simulink model "DynamicTemplate"  (R2018b)
settings: Solver=FixedStepDiscrete  StartTime=0.0  StopTime=Inf  FixedStep=0.001  RelTol=1e-3  EnableMultiTasking=on
undefined symbols (not defined in the file): J1, J2, J3, J4, J5, J6, J7, Motor_Current, Motor_Position, Motor_Velocity, Send_GUIdata
libraries: c280xlib x50, simulink x5, idelinklib_common x1
(part 1 of 5)
settings Model: ExtModeTrigDuration=8  Creator=Administrator  LastModifiedBy=Jeason
settings SolverCC: AutoInsertRateTranBlk=on
settings OptimizationCC: DefaultUnderspecifiedDataType=single  EnhancedBackFolding=on  PassReuseOutputArgsAs=Individual arguments  MaxStackSize=512  OptimizeBlockOrder=speed  DifferentSizesBufferReuse=on  OptimizationCustomize=off
settings DebuggingCC: InheritedTsInSrcMsg=none  MultiTaskDSMMsg=none  ParameterTunabilityLossMsg=error
settings HardwareCC: ProdBitPerChar=16  ProdBitPerInt=16  ProdBitPerPointer=32  ProdBitPerSizeT=32  ProdBitPerPtrDiffT=32  ProdLargestAtomicInteger=Integer  ProdLargestAtomicFloat=None  ProdWordSize=16  ProdLongLongMode=on  ProdHWDeviceType=Texas Instruments->C2000
settings SFSimCC: MATLABDynamicMemAlloc=off
settings RTWCC: SystemTargetFile=ert.tlc  HardwareBoard=TI Delfino F2833x  TemplateMakefile=ert_default_tmf  GenerateReport=on  Toolchain=Texas Instruments Code Composer Studio (C2000)  IncludeHyperlinkInReport=on  LaunchReport=on  GenerateTraceInfo=on  GenerateTraceReport=on  GenerateTraceReportSl=on  GenerateTraceReportSf=on  GenerateTraceReportEml=on
settings CodeAppCC: ForceParamTrailComments=on  IgnoreCustomStorageClasses=off  OperatorAnnotations=on  SimulinkDataObjDesc=on  SFDataObjDesc=on  InsertBlockDesc=on
settings ERTTargetCC: CodeReplacementLibrary=TI C28x

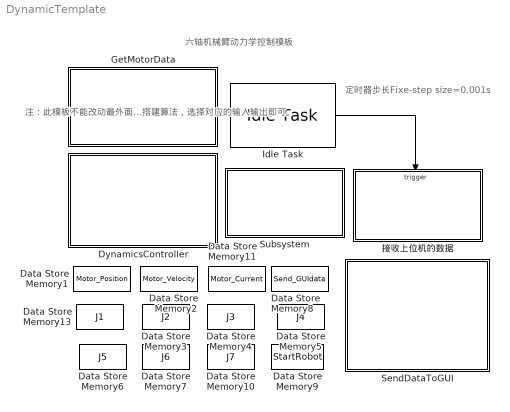
== system DynamicTemplate ==
  note: 六轴机械臂动力学控制模板
  note: 注：此模板不能改动最外面的结构，要做动力学算法只能在动力学计算子系统内部搭建算法，选择对应的输入输出即可。
  note: 定时器步长Fixe-step size=0.001s
  Data Store Memory1 : DataStoreMemory  DataStoreName=Motor_Position  ReadBeforeWriteMsg=warning  WriteAfterWriteMsg=warning  WriteAfterReadMsg=warning  InitialValue=[0 0 0 0 0 0]  ShowAdditionalParam=off  OutDataTypeStr=int32
      settings: RTWStateStorageClass=ExportedGlobal
  Data Store Memory10 : DataStoreMemory  DataStoreName=J7  ReadBeforeWriteMsg=warning  WriteAfterWriteMsg=warning  WriteAfterReadMsg=warning  InitialValue=[0 0 0 0 0 0]  ShowAdditionalParam=off  OutDataTypeStr=double
      settings: RTWStateStorageClass=ExportedGlobal
  Data Store Memory11 : DataStoreMemory  DataStoreName=Motor_Current  ReadBeforeWriteMsg=warning  WriteAfterWriteMsg=warning  WriteAfterReadMsg=warning  InitialValue=[0 0 0 0 0 0]  ShowAdditionalParam=off  OutDataTypeStr=int32
      settings: RTWStateStorageClass=ExportedGlobal
  Data Store Memory13 : DataStoreMemory  DataStoreName=J1  ReadBeforeWriteMsg=warning  WriteAfterWriteMsg=warning  WriteAfterReadMsg=warning  InitialValue=[0 0 0 0 0 0]  ShowAdditionalParam=off  OutDataTypeStr=double
      settings: RTWStateStorageClass=ExportedGlobal
  Data Store Memory2 : DataStoreMemory  DataStoreName=Motor_Velocity  ReadBeforeWriteMsg=warning  WriteAfterWriteMsg=warning  WriteAfterReadMsg=warning  InitialValue=[0 0 0 0 0 0]  ShowAdditionalParam=off  OutDataTypeStr=int32
      settings: RTWStateStorageClass=ExportedGlobal
  Data Store Memory3 : DataStoreMemory  DataStoreName=J2  ReadBeforeWriteMsg=warning  WriteAfterWriteMsg=warning  WriteAfterReadMsg=warning  InitialValue=[0 0 0 0 0 0]  ShowAdditionalParam=off  OutDataTypeStr=double
      settings: RTWStateStorageClass=ExportedGlobal
  Data Store Memory4 : DataStoreMemory  DataStoreName=J3  ReadBeforeWriteMsg=warning  WriteAfterWriteMsg=warning  WriteAfterReadMsg=warning  InitialValue=[0 0 0 0 0 0]  ShowAdditionalParam=off  OutDataTypeStr=double
      settings: RTWStateStorageClass=ExportedGlobal
  Data Store Memory5 : DataStoreMemory  DataStoreName=J4  ReadBeforeWriteMsg=warning  WriteAfterWriteMsg=warning  WriteAfterReadMsg=warning  InitialValue=[0 0 0 0 0 0]  ShowAdditionalParam=off  OutDataTypeStr=double
      settings: RTWStateStorageClass=ExportedGlobal
  Data Store Memory6 : DataStoreMemory  DataStoreName=J5  ReadBeforeWriteMsg=warning  WriteAfterWriteMsg=warning  WriteAfterReadMsg=warning  InitialValue=[0 0 0 0 0 0]  ShowAdditionalParam=off  OutDataTypeStr=double
      settings: RTWStateStorageClass=ExportedGlobal
  Data Store Memory7 : DataStoreMemory  DataStoreName=J6  ReadBeforeWriteMsg=warning  WriteAfterWriteMsg=warning  WriteAfterReadMsg=warning  InitialValue=[0 0 0 0 0 0]  ShowAdditionalParam=off  OutDataTypeStr=double
      settings: RTWStateStorageClass=ExportedGlobal
  Data Store Memory8 : DataStoreMemory  DataStoreName=Send_GUIdata  ReadBeforeWriteMsg=warning  WriteAfterWriteMsg=warning  WriteAfterReadMsg=warning  InitialValue=zeros(1,18)  ShowAdditionalParam=off  OutDataTypeStr=double
      settings: RTWStateStorageClass=ExportedGlobal
  Data Store Memory9 : DataStoreMemory  DataStoreName=StartRobot  ReadBeforeWriteMsg=warning  WriteAfterWriteMsg=warning  WriteAfterReadMsg=warning  ShowAdditionalParam=off  OutDataTypeStr=uint16
      settings: RTWStateStorageClass=ExportedGlobal
  DynamicsController : Subsystem  Tag=Calculated_Data  Priority=1  TreatAsAtomicUnit=on
      settings: RTWSystemCode=Nonreusable function  RTWFcnNameOpts=Use subsystem name  RTWFileNameOpts=Use subsystem name
      mask Display:
      | color('red')
      | disp('六轴机械臂动力学计算')
  GetMotorData : Subsystem  Tag=Get_Data  Priority=0  TreatAsAtomicUnit=on
      settings: RTWSystemCode=Nonreusable function
  Idle Task : idelinklib_common/Idle Task  tasknumbers=[0]  taskpriorities=100016  taskpreempts=[1]  showinput=off  simPriority=0
  SendDataToGUI : Subsystem  Priority=2  TreatAsAtomicUnit=on
      settings: RTWSystemCode=Nonreusable function
  Subsystem : Subsystem
      mask Display: disp('System\nInitialization');
  接收上位机的数据 : Subsystem  TreatAsAtomicUnit=on
  wires:
  Idle Task/1 -> 接收上位机的数据/Trigger

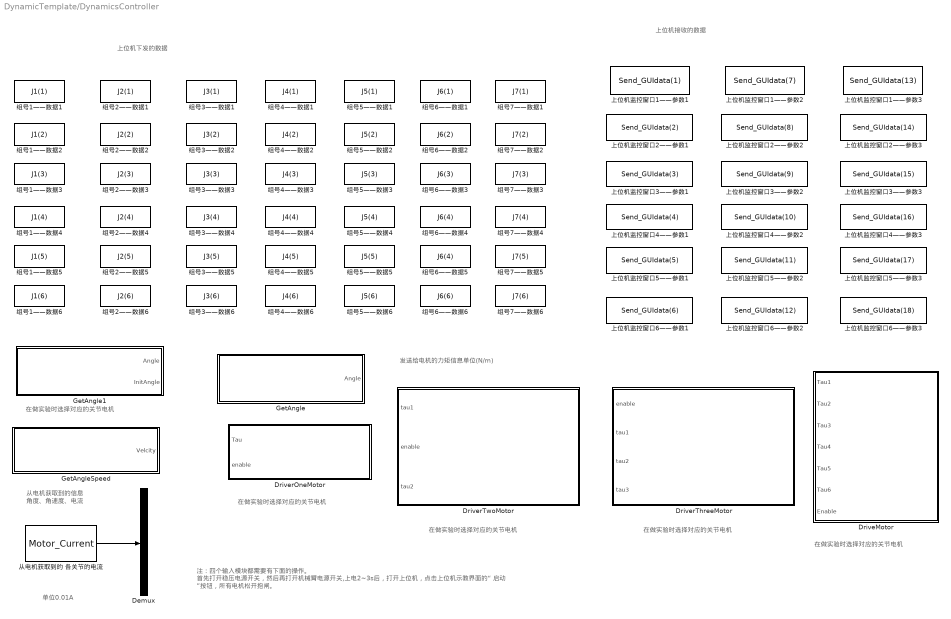
== system DynamicTemplate/DynamicsController ==
  note: 在做实验时选择对应的关节电机
  note: 在做实验时选择对应的关节电机
  note: 上位机接收的数据
  note: 单位0.01A
  note: 从电机获取到的信息
      | 角度、角速度、电流
  note: 注：四个输入模块都需要有下面的操作。
      | 首先打开稳压电源开关，然后再打开机械臂电源开关,上电2~3s后，打开上位机，点击上位机示教界面的“ 启动 ”按钮，所有电机松开抱闸。
  note: 在做实验时选择对应的关节电机
  note: 在做实验时选择对应的关节电机
  note: 在做实验时选择对应的关节电机
  note: 发送给电机的力矩信息单位(N/m)
  note: 上位机下发的数据
  Demux : Demux  Outputs=6
  DriveMotor : Subsystem  TreatAsAtomicUnit=on  RTWFcnName=DrivrMotor  mask(DriverMotor){Motor1=off, Motor2=off, Motor3=off, Motor4=off, Motor5=off, Motor6=off}
      mask help:
      | 当其中一个Motor勾选时，表示将力矩输出给对应的电机；如果不勾选时，表示对应的电机不工作。
      | 比如：如果做单关节实验时，哪个电机要做实验就勾选对应的电机，其他电机一定要不勾选。
      | 关节1~3为CANB,关节4~6为CANA,驱动邮箱号为7~12。输入量的范围限定在-900~900。
      mask init:
      | % 
      | %     vssBlk1 = [gcb, '/BottomDriver/Joint1'];
      | %     vssBlk2 = [gcb, '/BottomDriver/Joint2'];
      | %     vssBlk3 = [gcb, '/BottomDriver/Joint3'];
      | %     vssBlk4 = [gcb, '/BottomDriver/Joint4'];
      | %     vssBlk5 = [gcb, '/BottomDriver/Joint5'];
      | %     vssBlk6 = [gcb, '/BottomDriver/Joint6'];
      | %     choice1 = get_param(gcb,'Motor1');
      | %     choice2 = get_param(gcb,'Motor2');
      | %     choice3 = get_param(gcb,'Motor3');
      | %     choice4 = get_param(gcb,'Motor4');
      | %     choice5 = get_param(gcb,'Motor5');
      | %     choice6 = get_param(gcb,'Motor6');
      | %     if strcmp(choice1,'off')
      | %         set_param(vssBlk1, 'Commented','on');
      | %     else
      | %         set_param(vssBlk1, 'Commented','off');
      | %     end
      | %     if strcmp(choice2,'off')
      | %         set_param(vssBlk2, 'Commented','on');
      | %     else
      | %         set_param(vssBlk2, 'Commented','off');
      | %     end
      | %     if strcmp(choice3,'off')
      | %         set_param(vssBlk3, 'Commented','on');
      | %     else
      | %         set_param(vssBlk3, 'Commented','off');
      | %     end
      | %     if strcmp(choice4,'off')
      | %         set_param(vssBlk4, 'Commented','on');
      | %     else
      | %         set_param(vssBlk4, 'Commented','off');
      | %     end
      | %     if strcmp(choice5,'off')
      | %         set_param(vssBlk5, 'Commented','on');
      | %     else
      | %         set_param(vssBlk5, 'Commented','off');
      | %     end
      | %     if strcmp(choice6,'off')
      | %         set_param(vssBlk6, 'Commented','on');
      | %     else
      | %         set_param(vssBlk6, 'Commented','off');
      | %     end
      settings: RTWSystemCode=Nonreusable function  RTWFcnNameOpts=User specified  RTWFileNameOpts=Use function name  FunctionInterfaceSpec=Allow arguments  FunctionWithSeparateData=on
      mask Callback Motor1:
      | vssBlk1 = [gcb, '/BottomDriver/Joint1'];
      | choice1 = get_param(gcb,'Motor1');
      | if strcmp(choice1,'off')
      |         set_param(vssBlk1, 'Commented','on');
      |     else
      |         set_param(vssBlk1, 'Commented','off');
      | end
      | clear choice1 vssBlk1;
      mask Callback Motor2:
      | vssBlk2 = [gcb, '/BottomDriver/Joint2'];
      | choice2 = get_param(gcb,'Motor2');
      | if strcmp(choice2,'off')
      |         set_param(vssBlk2, 'Commented','on');
      |     else
      |         set_param(vssBlk2, 'Commented','off');
      | end
      | clear choice2 vssBlk2;
      mask Callback Motor3:
      | vssBlk3 = [gcb, '/BottomDriver/Joint3'];
      | choice3 = get_param(gcb,'Motor3');
      | if strcmp(choice3,'off')
      |         set_param(vssBlk3, 'Commented','on');
      |     else
      |         set_param(vssBlk3, 'Commented','off');
      | end
      | clear choice3 vssBlk3;
      mask Callback Motor4:
      | vssBlk4 = [gcb, '/BottomDriver/Joint4'];
      | choice4 = get_param(gcb,'Motor4');
      | if strcmp(choice4,'off')
      |         set_param(vssBlk4, 'Commented','on');
      |     else
      |         set_param(vssBlk4, 'Commented','off');
      | end
      | clear choice4 vssBlk4;
      mask Callback Motor5:
      | vssBlk5 = [gcb, '/BottomDriver/Joint5'];
      | choice5 = get_param(gcb,'Motor5');
      | if strcmp(choice5,'off')
      |         set_param(vssBlk5, 'Commented','on');
      |     else
      |         set_param(vssBlk5, 'Commented','off');
      | end
      | clear choice5 vssBlk5;
      mask Callback Motor6:
      | vssBlk6 = [gcb, '/BottomDriver/Joint6'];
      | choice6 = get_param(gcb,'Motor6');
      | if strcmp(choice6,'off')
      |         set_param(vssBlk6, 'Commented','on');
      |     else
      |         set_param(vssBlk6, 'Commented','off');
      | end
      | clear choice6 vssBlk6;
      mask Display:
      | disp('DriverMotor');
      | port_label('input', 1, 'Tau1');
      | port_label('input', 2, 'Tau2');
      | port_label('input', 3, 'Tau3');
      | port_label('input', 4, 'Tau4');
      | port_label('input', 5, 'Tau5');
      | port_label('input', 6, 'Tau6');
      | port_label('input', 7, 'Enable');
  DriverOneMotor : Subsystem  TreatAsAtomicUnit=on  RTWFcnName=DriverOneMotor  mask(驱动单个关节){SelectJoint=1}
      mask prompts: SelectJoint "选择关节电机"
      mask help:
      | 关节1~3为CANB,关节4~6为CANA,驱动的电机的邮箱号统一为7。
      | 输入量的范围限定在-900~900。
      settings: RTWSystemCode=Nonreusable function  RTWFcnNameOpts=User specified  RTWFileNameOpts=Use function name  FunctionInterfaceSpec=Allow arguments  FunctionWithSeparateData=on
      mask TypeOptions SelectJoint: 1 | 2 | 3 | 4 | 5 | 6
      mask Callback SelectJoint:
      | vssBlk1_1 = [gcb, '/BottomDriver/Joint1'];
      | vssBlk1_2 = [gcb, '/BottomDriver/Joint2'];
      | vssBlk1_3 = [gcb, '/BottomDriver/Joint3'];
      | vssBlk1_4 = [gcb, '/BottomDriver/Joint4'];
      | vssBlk1_5 = [gcb, '/BottomDriver/Joint5'];
      | vssBlk1_6 = [gcb, '/BottomDriver/Joint6'];
      | choice1 = get_param(gcb,'SelectJoint');
      | if strcmp(choice1,'1')
      |     set_param(vssBlk1_1, 'Commented','off');
      |     set_param(vssBlk1_2,'Commented','on');
      |     set_param(vssBlk1_3,'Commented','on');
      |     set_param(vssBlk1_4,'Commented','on');
      |     set_param(vssBlk1_5,'Commented','on');
      |     set_param(vssBlk1_6,'Commented','on');
      | elseif strcmp(choice1,'2')
      |     set_param(vssBlk1_2, 'Commented','off');
      |     set_param(vssBlk1_1,'Commented','on');
      |     set_param(vssBlk1_3,'Commented','on');
      |     set_param(vssBlk1_4,'Commented','on');
      |     set_param(vssBlk1_5,'Commented','on');
      |     set_param(vssBlk1_6,'Commented','on');
      | elseif strcmp(choice1,'3')
      |     set_param(vssBlk1_3, 'Commented','off');
      |     set_param(vssBlk1_1,'Commented','on');
      |     set_param(vssBlk1_2,'Commented','on');
      |     set_param(vssBlk1_4,'Commented','on');
      |     set_param(vssBlk1_5,'Commented','on');
      |     set_param(vssBlk1_6,'Commented','on');
      | elseif strcmp(choice1,'4')
      |     set_param(vssBlk1_4, 'Commented','off');
      |     set_param(vssBlk1_1,'Commented','on');
      |     set_param(vssBlk1_2,'Commented','on');
      |     set_param(vssBlk1_3,'Commented','on');
      |     set_param(vssBlk1_5,'Commented','on');
      |     set_param(vssBlk1_6,'Commented','on');
      | elseif strcmp(choice1,'5')
      |     set_param(vssBlk1_5, 'Commented','off');
      |     set_param(vssBlk1_1,'Commented','on');
      |     set_param(vssBlk1_2,'Commented','on');
      |     set_param(vssBlk1_3,'Commented','on');
      |     set_param(vssBlk1_4,'Commented','on');
      |     set_param(vssBlk1_6,'Commented','on');
      | elseif strcmp(choice1,'6')
      |     set_param(vssBlk1_6, 'Commented','off');
      |     set_param(vssBlk1_1,'Commented','on');
      |     set_param(vssBlk1_2,'Commented','on');
      |     set_param(vssBlk1_3,'Commented','on');
      |     set_param(vssBlk1_4,'Commented','on');
      |     set_param(vssBlk1_5,'Commented','on');
      | end
      | clear choice1 vssBlk1_1 vssBlk1_2 vssBlk1_3 vssBlk1_4 vssBlk1_5 vssBlk1_6;
      mask Display:
      | port_label('input', 1, 'Tau');
      | port_label('input', 2, 'Enable');
      | choice1 = get_param(gcb,'SelectJoint');
      | color('black');
      | switch choice1
      |     case '1'
      |         disp('单关节算法\n驱动关节1电机');
      |     case '2'
      |         disp('单关节算法\n驱动关节2电机');
      |     case '3'
      |         disp('单关节算法\n驱动关节3电机');
      |     case '4'
      |         disp('单关节算法\n驱动关节4电机');
      |     case '5'
      |         disp('单关节算法\n驱动关节5电机');
      |     case '6'
      |         disp('单关节算法\n驱动关节6电机');
      | end
      | clear choice1;
  DriverThreeMotor : Subsystem  TreatAsAtomicUnit=on  RTWFcnName=DriverThreeMotor  mask(驱动三个关节){SelectJoint1=1, SelectJoint2=2, SelectJoint3=3}
      mask prompts: SelectJoint1 "选择关节电机1"; SelectJoint2 "选择关节电机2"; SelectJoint3 "选择关节电机3"
      mask help:
      | 关节1~3为CANB,关节4~6为CANA,驱动的第一个电机的邮箱号为7，驱动的第二个电机电机的邮箱号为8，驱动的第二个电机电机的邮箱号为9。
      | 输入量的范围限定在-900~900。
      mask init:
      | vssBlk1_1 = [gcb, '/BottomDriver/Judgement/OneJoint/Joint1'];
      | vssBlk1_2 = [gcb, '/BottomDriver/Judgement/OneJoint/Joint2'];
      | vssBlk1_3 = [gcb, '/BottomDriver/Judgement/OneJoint/Joint3'];
      | vssBlk1_4 = [gcb, '/BottomDriver/Judgement/OneJoint/Joint4'];
      | vssBlk1_5 = [gcb, '/BottomDriver/Judgement/OneJoint/Joint5'];
      | vssBlk1_6 = [gcb, '/BottomDriver/Judgement/OneJoint/Joint6'];
      | vssBlk2_1 = [gcb, '/BottomDriver/Judgement/TwoJoint/Joint1'];
      | vssBlk2_2 = [gcb, '/BottomDriver/Judgement/TwoJoint/Joint2'];
      | vssBlk2_3 = [gcb, '/BottomDriver/Judgement/TwoJoint/Joint3'];
      | vssBlk2_4 = [gcb, '/BottomDriver/Judgement/TwoJoint/Joint4'];
      | vssBlk2_5 = [gcb, '/BottomDriver/Judgement/TwoJoint/Joint5'];
      | vssBlk2_6 = [gcb, '/BottomDriver/Judgement/TwoJoint/Joint6'];
      | vssBlk3_1 = [gcb, '/BottomDriver/Judgement/ThreeJoint/Joint1'];
      | vssBlk3_2 = [gcb, '/BottomDriver/Judgement/ThreeJoint/Joint2'];
      | vssBlk3_3 = [gcb, '/BottomDriver/Judgement/ThreeJoint/Joint3'];
      | vssBlk3_4 = [gcb, '/BottomDriver/Judgement/ThreeJoint/Joint4'];
      | vssBlk3_5 = [gcb, '/BottomDriver/Judgement/ThreeJoint/Joint5'];
      | vssBlk3_6 = [gcb, '/BottomDriver/Judgement/ThreeJoint/Joint6'];
      | choice1 = get_param(gcb,'SelectJoint1');
      | choice2 = get_param(gcb,'SelectJoint2');
      | choice3 = get_param(gcb,'SelectJoint3');
      | if ((strcmp(choice1,'1'))&&(strcmp(choice2,'1')))||((strcmp(choice1,'1'))&&(strcmp(choice3,'1')))||(((strcmp(choice2,'1'))&&(strcmp(choice3,'1'))))
      |     error('Error. Input can not be the same.');
      | end
      | if ((strcmp(choice1,'2'))&&(strcmp(choice2,'2')))||((strcmp(choice1,'2'))&&(strcmp(choice3,'2')))||(((strcmp(choice2,'2'))&&(strcmp(choice3,'2'))))
      |     error('Error. Input can not be the same.');
      | end
      | if ((strcmp(choice1,'3'))&&(strcmp(choice2,'3')))||((strcmp(choice1,'3'))&&(strcmp(choice3,'3')))||(((strcmp(choice2,'3'))&&(strcmp(choice3,'3'))))
      |     error('Error. Input can not be the same.');
      | end
      | if ((strcmp(choice1,'4'))&&(strcmp(choice2,'4')))||((strcmp(choice1,'4'))&&(strcmp(choice3,'4')))||(((strcmp(choice2,'4'))&&(strcmp(choice3,'4'))))
      |     error('Error. Input can not be the same.');
      | end
      | if ((strcmp(choice1,'5'))&&(strcmp(choice2,'5')))||((strcmp(choice1,'5'))&&(strcmp(choice3,'5')))||(((strcmp(choice2,'5'))&&(strcmp(choice3,'5'))))
      |     error('Error. Input can not be the same.');
      | end
      | if ((strcmp(choice1,'6'))&&(strcmp(choice2,'6')))||((strcmp(choice1,'6'))&&(strcmp(choice3,'6')))||(((strcmp(choice2,'6'))&&(strcmp(choice3,'6'))))
      |     error('Error. Input can not be the same.');
      | end
      | clear choice1 vssBlk1_1 vssBlk1_2 vssBlk1_3 vssBlk1_4 vssBlk1_5 vssBlk1_6; 
      | clear choice2 vssBlk2_1 vssBlk2_2 vssBlk2_3 vssBlk2_4 vssBlk2_5 vssBlk2_6; 
      | clear choice3 vssBlk3_1 vssBlk3_2 vssBlk3_3 vssBlk3_4 vssBlk3_5 vssBlk3_6;
      settings: RTWSystemCode=Nonreusable function  RTWFcnNameOpts=User specified  RTWFileNameOpts=Use function name  FunctionInterfaceSpec=Allow arguments  FunctionWithSeparateData=on
      mask TypeOptions SelectJoint1: 1 | 2 | 3 | 4 | 5 | 6
      mask Callback SelectJoint1:
      | vssBlk1_1 = [gcb, '/BottomDriver/Judgement/OneJoint/Joint1'];
      |     vssBlk1_2 = [gcb, '/BottomDriver/Judgement/OneJoint/Joint2'];
      |     vssBlk1_3 = [gcb, '/BottomDriver/Judgement/OneJoint/Joint3'];
      |     vssBlk1_4 = [gcb, '/BottomDriver/Judgement/OneJoint/Joint4'];
      |     vssBlk1_5 = [gcb, '/BottomDriver/Judgement/OneJoint/Joint5'];
      |     vssBlk1_6 = [gcb, '/BottomDriver/Judgement/OneJoint/Joint6'];
      |     choice1 = get_param(gcb,'SelectJoint1');
      |     if strcmp(choice1,'1')
      |         set_param(vssBlk1_1, 'Commented','off');
      |         set_param(vssBlk1_2,'Commented','on');
      |         set_param(vssBlk1_3,'Commented','on');
      |         set_param(vssBlk1_4,'Commented','on');
      |         set_param(vssBlk1_5,'Commented','on');
      |         set_param(vssBlk1_6,'Commented','on');
      |     elseif strcmp(choice1,'2')
      |         set_param(vssBlk1_2, 'Commented','off');
      |         set_param(vssBlk1_1,'Commented','on');
      |         set_param(vssBlk1_3,'Commented','on');
      |         set_param(vssBlk1_4,'Commented','on');
      |         set_param(vssBlk1_5,'Commented','on');
      |         set_param(vssBlk1_6,'Commented','on');
      |     elseif strcmp(choice1,'3')
      |         set_param(vssBlk1_3, 'Commented','off');
      |         set_param(vssBlk1_1,'Commented','on');
      |         set_param(vssBlk1_2,'Commented','on');
      |         set_param(vssBlk1_4,'Commented','on');
      |         set_param(vssBlk1_5,'Commented','on');
      |         set_param(vssBlk1_6,'Commented','on');
      |     elseif strcmp(choice1,'4')
      |         set_param(vssBlk1_4, 'Commented','off');
      |         set_param(vssBlk1_1,'Commented','on');
      |         set_param(vssBlk1_2,'Commented','on');
      |         set_param(vssBlk1_3,'Commented','on');
      |         set_param(vssBlk1_5,'Commented','on');
      |         set_param(vssBlk1_6,'Commented','on');
      |     elseif strcmp(choice1,'5')
      |         set_param(vssBlk1_5, 'Commented','off');
      |         set_param(vssBlk1_1,'Commented','on');
      |         set_param(vssBlk1_2,'Commented','on');
      |         set_param(vssBlk1_3,'Commented','on');
      |         set_param(vssBlk1_4,'Commented','on');
      |         set_param(vssBlk1_6,'Commented','on');
      |     elseif strcmp(choice1,'6')
      |         set_param(vssBlk1_6, 'Commented','off');
      |         set_param(vssBlk1_1,'Commented','on');
      |         set_param(vssBlk1_2,'Commented','on');
      |         set_param(vssBlk1_3,'Commented','on');
      |         set_param(vssBlk1_4,'Commented','on');
      |         set_param(vssBlk1_5,'Commented','on');
      |     end
      |     clear choice1 vssBlk1_1 vssBlk1_2 vssBlk1_3 vssBlk1_4 vssBlk1_5 vssBlk1_6;
      mask TypeOptions SelectJoint2: 1 | 2 | 3 | 4 | 5 | 6
      mask Callback SelectJoint2:
      | vssBlk2_1 = [gcb, '/BottomDriver/Judgement/TwoJoint/Joint1'];
      |     vssBlk2_2 = [gcb, '/BottomDriver/Judgement/TwoJoint/Joint2'];
      |     vssBlk2_3 = [gcb, '/BottomDriver/Judgement/TwoJoint/Joint3'];
      |     vssBlk2_4 = [gcb, '/BottomDriver/Judgement/TwoJoint/Joint4'];
      |     vssBlk2_5 = [gcb, '/BottomDriver/Judgement/TwoJoint/Joint5'];
      |     vssBlk2_6 = [gcb, '/BottomDriver/Judgement/TwoJoint/Joint6'];
      |     choice2 = get_param(gcb,'SelectJoint2');
      |      if strcmp(choice2,'1')
      |         set_param(vssBlk2_1, 'Commented','off');
      |         set_param(vssBlk2_2,'Commented','on');
      |         set_param(vssBlk2_3,'Commented','on');
      |         set_param(vssBlk2_4,'Commented','on');
      |         set_param(vssBlk2_5,'Commented','on');
      |         set_param(vssBlk2_6,'Commented','on');
      |     elseif strcmp(choice2,'2')
      |         set_param(vssBlk2_2, 'Commented','off');
      |         set_param(vssBlk2_1,'Commented','on');
      |         set_param(vssBlk2_3,'Commented','on');
      |         set_param(vssBlk2_4,'Commented','on');
      |         set_param(vssBlk2_5,'Commented','on');
      |         set_param(vssBlk2_6,'Commented','on');
      |     elseif strcmp(choice2,'3')
      |         set_param(vssBlk2_3, 'Commented','off');
      |         set_param(vssBlk2_1,'Commented','on');
      |         set_param(vssBlk2_2,'Commented','on');
      |         set_param(vssBlk2_4,'Commented','on');
      |         set_param(vssBlk2_5,'Commented','on');
      |         set_param(vssBlk2_6,'Commented','on');
      |     elseif strcmp(choice2,'4')
      |         set_param(vssBlk2_4, 'Commented','off');
      |         set_param(vssBlk2_1,'Commented','on');
      |         set_param(vssBlk2_2,'Commented','on');
      |         set_param(vssBlk2_3,'Commented','on');
      |         set_param(vssBlk2_5,'Commented','on');
      |         set_param(vssBlk2_6,'Commented','on');
      |     elseif strcmp(choice2,'5')
      |         set_param(vssBlk2_5, 'Commented','off');
      |         set_param(vssBlk2_1,'Commented','on');
      |         set_param(vssBlk2_2,'Commented','on');
      |         set_param(vssBlk2_3,'Commented','on');
      |         set_param(vssBlk2_4,'Commented','on');
      |         set_param(vssBlk2_6,'Commented','on');
      |     elseif strcmp(choice2,'6')
      |         set_param(vssBlk2_6, 'Commented','off');
      |         set_param(vssBlk2_1,'Commented','on');
      |         set_param(vssBlk2_2,'Commented','on');
      |         set_param(vssBlk2_3,'Commented','on');
      |         set_param(vssBlk2_4,'Commented','on');
      |         set_param(vssBlk2_5,'Commented','on');
      |      end
      |     clear choice2 vssBlk2_1 vssBlk2_2 vssBlk2_3 vssBlk2_4 vssBlk2_5 vssBlk2_6;
      mask TypeOptions SelectJoint3: 1 | 2 | 3 | 4 | 5 | 6
      mask Callback SelectJoint3:
      | vssBlk3_1 = [gcb, '/BottomDriver/Judgement/ThreeJoint/Joint1'];
      |     vssBlk3_2 = [gcb, '/BottomDriver/Judgement/ThreeJoint/Joint2'];
      |     vssBlk3_3 = [gcb, '/BottomDriver/Judgement/ThreeJoint/Joint3'];
      |     vssBlk3_4 = [gcb, '/BottomDriver/Judgement/ThreeJoint/Joint4'];
      |     vssBlk3_5 = [gcb, '/BottomDriver/Judgement/ThreeJoint/Joint5'];
      |     vssBlk3_6 = [gcb, '/BottomDriver/Judgement/ThreeJoint/Joint6'];
      |     choice3 = get_param(gcb,'SelectJoint3');
      |     if strcmp(choice3,'1')
      |         set_param(vssBlk3_1, 'Commented','off');
      |         set_param(vssBlk3_2,'Commented','on');
      |         set_param(vssBlk3_3,'Commented','on');
      |         set_param(vssBlk3_4,'Commented','on');
      |         set_param(vssBlk3_5,'Commented','on');
      |         set_param(vssBlk3_6,'Commented','on');
      |     elseif strcmp(choice3,'2')
      |         set_param(vssBlk3_2, 'Commented','off');
      |         set_param(vssBlk3_1,'Commented','on');
      |         set_param(vssBlk3_3,'Commented','on');
      |         set_param(vssBlk3_4,'Commented','on');
      |         set_param(vssBlk3_5,'Commented','on');
      |         set_param(vssBlk3_6,'Commented','on');
      |     elseif strcmp(choice3,'3')
      |         set_param(vssBlk3_3, 'Commented','off');
      |         set_param(vssBlk3_1,'Commented','on');
      |         set_param(vssBlk3_2,'Commented','on');
      |         set_param(vssBlk3_4,'Commented','on');
      |         set_param(vssBlk3_5,'Commented','on');
      |         set_param(vssBlk3_6,'Commented','on');
      |     elseif strcmp(choice3,'4')
      |         set_param(vssBlk3_4, 'Commented','off');
      |         set_param(vssBlk3_1,'Commented','on');
      |         set_param(vssBlk3_2,'Commented','on');
      |         set_param(vssBlk3_3,'Commented','on');
      |         set_param(vssBlk3_5,'Commented','on');
      |         set_param(vssBlk3_6,'Commented','on');
      |     elseif strcmp(choice3,'5')
      |         set_param(vssBlk3_5, 'Commented','off');
      |         set_param(vssBlk3_1,'Commented','on');
      |         set_param(vssBlk3_2,'Commented','on');
      |         set_param(vssBlk3_3,'Commented','on');
      |         set_param(vssBlk3_4,'Commented','on');
      |         set_param(vssBlk3_6,'Commented','on');
      |     elseif strcmp(choice3,'6')
      |         set_param(vssBlk3_6, 'Commented','off');
      |         set_param(vssBlk3_1,'Commented','on');
      |         set_param(vssBlk3_2,'Commented','on');
      |         set_param(vssBlk3_3,'Commented','on');
      |         set_param(vssBlk3_4,'Commented','on');
      |         set_param(vssBlk3_5,'Commented','on');
      |     end
      |     clear choice3 vssBlk3_1 vssBlk3_2 vssBlk3_3 vssBlk3_4 vssBlk3_5 vssBlk3_6;
      mask Display:
      | str1='三关节算法';str2='驱动关节'; str3='、';str4='、';str5='电机';
      | choice1 = get_param(gcb,'SelectJoint1');
      | choice2 = get_param(gcb,'SelectJoint2');
      | choice3 = get_param(gcb,'SelectJoint3');
      | str=[str1,'\n',str2,choice1,str3,choice2,str4,choice3,str5];
      | disp(str);
      | port_label('input', 1, 'Enable');
      | port_label('input', 2, 'Tau1');
      | port_label('input', 3, 'Tau2');
      | port_label('input', 4, 'Tau3');
      | clear str str1 str2 str3 str4 str5 choice1 choice2 choice3；
  DriverTwoMotor : Subsystem  TreatAsAtomicUnit=on  RTWFcnName=DriverTwoMotor  mask(驱动两个关节){SelectJoint1=1, SelectJoint2=2}
      mask prompts: SelectJoint1 "选择关节电机1"; SelectJoint2 "选择关节电机2"
      mask help:
      | 关节1~3为CANB,关节4~6为CANA,驱动的第一个电机的邮箱号为7，驱动的第二个电机的邮箱号为8。
      | 输入量的范围限定在-900~900。
      mask init:
      | vssBlk1_1 = [gcb, '/BottomDriver/Judgement/OneJoint/Joint1'];
      |     vssBlk1_2 = [gcb, '/BottomDriver/Judgement/OneJoint/Joint2'];
      |     vssBlk1_3 = [gcb, '/BottomDriver/Judgement/OneJoint/Joint3'];
      |     vssBlk1_4 = [gcb, '/BottomDriver/Judgement/OneJoint/Joint4'];
      |     vssBlk1_5 = [gcb, '/BottomDriver/Judgement/OneJoint/Joint5'];
      |     vssBlk1_6 = [gcb, '/BottomDriver/Judgement/OneJoint/Joint6'];
      |     vssBlk2_1 = [gcb, '/BottomDriver/Judgement/TwoJoint/Joint1'];
      |     vssBlk2_2 = [gcb, '/BottomDriver/Judgement/TwoJoint/Joint2'];
      |     vssBlk2_3 = [gcb, '/BottomDriver/Judgement/TwoJoint/Joint3'];
      |     vssBlk2_4 = [gcb, '/BottomDriver/Judgement/TwoJoint/Joint4'];
      |     vssBlk2_5 = [gcb, '/BottomDriver/Judgement/TwoJoint/Joint5'];
      |     vssBlk2_6 = [gcb, '/BottomDriver/Judgement/TwoJoint/Joint6'];
      |     choice1 = get_param(gcb,'SelectJoint1');
      |     choice2 = get_param(gcb,'SelectJoint2');
      |     if (strcmp(choice1,'1'))&&(strcmp(choice2,'1'))
      |         error('Error. Input can not be the same.');
      |     end
      |     if (strcmp(choice1,'2'))&&(strcmp(choice2,'2'))
      |         error('Error. Input can not be the same.');
      |     end
      |     if (strcmp(choice1,'3'))&&(strcmp(choice2,'3'))
      |         error('Error. Input can not be the same.');
      |     end
      |     if (strcmp(choice1,'4'))&&(strcmp(choice2,'4'))
      |         error('Error. Input can not be the same.');
      |     end
      |     if (strcmp(choice1,'5'))&&(strcmp(choice2,'5'))
      |         error('Error. Input can not be the same.');
      |     end
      |     if (strcmp(choice1,'6'))&&(strcmp(choice2,'6'))
      |         error('Error. Input can not be the same.');
      |     end
      |     clear choice1 vssBlk1_1 vssBlk1_2 vssBlk1_3 vssBlk1_4 vssBlk1_5 vssBlk1_6; 
      |     clear choice2 vssBlk2_1 vssBlk2_2 vssBlk2_3 vssBlk2_4 vssBlk2_5 vssBlk2_6;
      settings: RTWSystemCode=Nonreusable function  RTWFcnNameOpts=User specified  RTWFileNameOpts=Use function name  FunctionInterfaceSpec=Allow arguments  FunctionWithSeparateData=on
      mask TypeOptions SelectJoint1: 1 | 2 | 3 | 4 | 5 | 6
      mask Callback SelectJoint1:
      | vssBlk1_1 = [gcb, '/BottomDriver/Judgement/OneJoint/Joint1'];
      | vssBlk1_2 = [gcb, '/BottomDriver/Judgement/OneJoint/Joint2'];
      | vssBlk1_3 = [gcb, '/BottomDriver/Judgement/OneJoint/Joint3'];
      | vssBlk1_4 = [gcb, '/BottomDriver/Judgement/OneJoint/Joint4'];
      | vssBlk1_5 = [gcb, '/BottomDriver/Judgement/OneJoint/Joint5'];
      | vssBlk1_6 = [gcb, '/BottomDriver/Judgement/OneJoint/Joint6'];
      | choice1 = get_param(gcb,'SelectJoint1');
      | if strcmp(choice1,'1')
      |     set_param(vssBlk1_1, 'Commented','off');
      |     set_param(vssBlk1_2,'Commented','on');
      |     set_param(vssBlk1_3,'Commented','on');
      |     set_param(vssBlk1_4,'Commented','on');
      |     set_param(vssBlk1_5,'Commented','on');
      |     set_param(vssBlk1_6,'Commented','on');
      | elseif strcmp(choice1,'2')
      |     set_param(vssBlk1_2, 'Commented','off');
      |     set_param(vssBlk1_1,'Commented','on');
      |     set_param(vssBlk1_3,'Commented','on');
      |     set_param(vssBlk1_4,'Commented','on');
      |     set_param(vssBlk1_5,'Commented','on');
      |     set_param(vssBlk1_6,'Commented','on');
      | elseif strcmp(choice1,'3')
      |     set_param(vssBlk1_3, 'Commented','off');
      |     set_param(vssBlk1_1,'Commented','on');
      |     set_param(vssBlk1_2,'Commented','on');
      |     set_param(vssBlk1_4,'Commented','on');
      |     set_param(vssBlk1_5,'Commented','on');
      |     set_param(vssBlk1_6,'Commented','on');
      | elseif strcmp(choice1,'4')
      |     set_param(vssBlk1_4, 'Commented','off');
      |     set_param(vssBlk1_1,'Commented','on');
      |     set_param(vssBlk1_2,'Commented','on');
      |     set_param(vssBlk1_3,'Commented','on');
      |     set_param(vssBlk1_5,'Commented','on');
      |     set_param(vssBlk1_6,'Commented','on');
      | elseif strcmp(choice1,'5')
      |     set_param(vssBlk1_5, 'Commented','off');
      |     set_param(vssBlk1_1,'Commented','on');
      |     set_param(vssBlk1_2,'Commented','on');
      |     set_param(vssBlk1_3,'Commented','on');
      |     set_param(vssBlk1_4,'Commented','on');
      |     set_param(vssBlk1_6,'Commented','on');
      | elseif strcmp(choice1,'6')
      |     set_param(vssBlk1_6, 'Commented','off');
      |     set_param(vssBlk1_1,'Commented','on');
      |     set_param(vssBlk1_2,'Commented','on');
      |     set_param(vssBlk1_3,'Commented','on');
      |     set_param(vssBlk1_4,'Commented','on');
      |     set_param(vssBlk1_5,'Commented','on');
      | end
      | clear choice1 vssBlk1_1 vssBlk1_2 vssBlk1_3 vssBlk1_4 vssBlk1_5 vssBlk1_6;
      mask TypeOptions SelectJoint2: 1 | 2 | 3 | 4 | 5 | 6
      mask Callback SelectJoint2:
      | vssBlk2_1 = [gcb, '/BottomDriver/Judgement/TwoJoint/Joint1'];
      | vssBlk2_2 = [gcb, '/BottomDriver/Judgement/TwoJoint/Joint2'];
      | vssBlk2_3 = [gcb, '/BottomDriver/Judgement/TwoJoint/Joint3'];
      | vssBlk2_4 = [gcb, '/BottomDriver/Judgement/TwoJoint/Joint4'];
      | vssBlk2_5 = [gcb, '/BottomDriver/Judgement/TwoJoint/Joint5'];
      | vssBlk2_6 = [gcb, '/BottomDriver/Judgement/TwoJoint/Joint6'];
      | choice2 = get_param(gcb,'SelectJoint2');
      |  if strcmp(choice2,'1')
      |     set_param(vssBlk2_1, 'Commented','off');
      |     set_param(vssBlk2_2,'Commented','on');
      |     set_param(vssBlk2_3,'Commented','on');
      |     set_param(vssBlk2_4,'Commented','on');
      |     set_param(vssBlk2_5,'Commented','on');
      |     set_param(vssBlk2_6,'Commented','on');
      | elseif strcmp(choice2,'2')
      |     set_param(vssBlk2_2, 'Commented','off');
      |     set_param(vssBlk2_1,'Commented','on');
      |     set_param(vssBlk2_3,'Commented','on');
      |     set_param(vssBlk2_4,'Commented','on');
      |     set_param(vssBlk2_5,'Commented','on');
      |     set_param(vssBlk2_6,'Commented','on');
      | elseif strcmp(choice2,'3')
      |     set_param(vssBlk2_3, 'Commented','off');
      |     set_param(vssBlk2_1,'Commented','on');
      |     set_param(vssBlk2_2,'Commented','on');
      |     set_param(vssBlk2_4,'Commented','on');
      |     set_param(vssBlk2_5,'Commented','on');
      |     set_param(vssBlk2_6,'Commented','on');
      | elseif strcmp(choice2,'4')
      |     set_param(vssBlk2_4, 'Commented','off');
      |     set_param(vssBlk2_1,'Commented','on');
      |     set_param(vssBlk2_2,'Commented','on');
      |     set_param(vssBlk2_3,'Commented','on');
      |     set_param(vssBlk2_5,'Commented','on');
      |     set_param(vssBlk2_6,'Commented','on');
      | elseif strcmp(choice2,'5')
      |     set_param(vssBlk2_5, 'Commented','off');
      |     set_param(vssBlk2_1,'Commented','on');
      |     set_param(vssBlk2_2,'Commented','on');
      |     set_param(vssBlk2_3,'Commented','on');
      |     set_param(vssBlk2_4,'Commented','on');
      |     set_param(vssBlk2_6,'Commented','on');
      | elseif strcmp(choice2,'6')
      |     set_param(vssBlk2_6, 'Commented','off');
      |     set_param(vssBlk2_1,'Commented','on');
      |     set_param(vssBlk2_2,'Commented','on');
      |     set_param(vssBlk2_3,'Commented','on');
      |     set_param(vssBlk2_4,'Commented','on');
      |     set_param(vssBlk2_5,'Commented','on');
      | end
      | clear choice2 vssBlk2_1 vssBlk2_2 vssBlk2_3 vssBlk2_4 vssBlk2_5 vssBlk2_6;
      mask Display:
      | str1='双关节算法';str2='驱动关节'; str3='和';str4='电机';
      | choice1 = get_param(gcb,'SelectJoint1');
      | choice2 = get_param(gcb,'SelectJoint2');
      | str=[str1,'\n',str2,choice1,str3,choice2,str4];
      | disp(str);
      | port_label('input', 1, 'Tau1');
      | port_label('input', 2, 'Enable');
      | port_label('input', 3, 'Tau2');
  GetAngle : Subsystem  TreatAsAtomicUnit=on  mask(获取电机外转子角度(rad)){JJoint=3, InitAngle=0}
      mask prompts: JJoint "选择关节电机"; InitAngle "给定初始角度(deg)"
      mask help:
      | 给定初始角度：假设在数学建模时，设定连杆在水平位置为0°，而机械臂每个关节在出厂时都设定在竖直位置为0°，那么这里就需要给定一个偏置值90°/-90°，默认设为0。
      | 注：关节3因为结构原因实际获取到的角度的正负和标签贴的方向相反。
      | Angle(rad)=电机外转子的实际角度值-给定的初始角度值
      mask TypeOptions JJoint: 1 | 2 | 3 | 4 | 5 | 6
      mask Display:
      | choice1 = get_param(gcb,'JJoint');
      | color('black');
      | switch choice1
      |     case '1'
      |         disp('获取关节1电机\n外转子角度(rad)');
      |     case '2'
      |         disp('获取关节2电机\n外转子角度(rad)');
      |     case '3'
      |         disp('获取关节3电机\n外转子角度(rad)');
      |     case '4'
      |         disp('获取关节4电机\n外转子角度(rad)');
      |     case '5'
      |         disp('获取关节5电机\n外转子角度(rad)');
      |     case '6'
      |         disp('获取关节6电机\n外转子角度(rad)');
      | end
      | color('black');
      | port_label('output', 1, 'Angle');
      | clear choice1;
  GetAngle1 : Subsystem  TreatAsAtomicUnit=on  mask(获取电机外转子角度(rad)){JJoint=3, InitAngle=0}
      mask prompts: JJoint "选择关节电机"; InitAngle "给定初始角度(deg)"
      mask help:
      | 给定初始角度：假设在数学建模时，设定连杆在水平位置为0°，而机械臂每个关节在出厂时都设定在竖直位置为0°，那么这里就需要给定一个偏置值90°/-90°，默认设为0。
      | 注：关节3因为结构原因实际获取到的角度的正负和标签贴的方向相反。
      | Angle(rad)=电机外转子的实际角度值-给定的初始角度值
      | InitAngle(rad)=给定的初始角度值
      mask TypeOptions JJoint: 1 | 2 | 3 | 4 | 5 | 6
      mask Display:
      | choice1 = get_param(gcb,'JJoint');
      | color('black');
      | switch choice1
      |     case '1'
      |         disp('获取关节1电机\n外转子角度(rad)');
      |     case '2'
      |         disp('获取关节2电机\n外转子角度(rad)');
      |     case '3'
      |         disp('获取关节3电机\n外转子角度(rad)');
      |     case '4'
      |         disp('获取关节4电机\n外转子角度(rad)');
      |     case '5'
      |         disp('获取关节5电机\n外转子角度(rad)');
      |     case '6'
      |         disp('获取关节6电机\n外转子角度(rad)');
      | end
      | color('black');
      | port_label('output', 1, 'Angle');
      | port_label('output', 2, 'InitAngle');
      | clear choice1;
  GetAngleSpeed : Subsystem  TreatAsAtomicUnit=on  mask{JJoint=3}
      mask prompts: JJoint "选择关节电机"
      mask help: 读取电机角速度(rad/s)
      mask TypeOptions JJoint: 1 | 2 | 3 | 4 | 5 | 6
      mask Display:
      | choice1 = get_param(gcb,'JJoint');
      | color('black');
      | switch choice1
      |     case '1'
      |         disp('获取关节1电机\n外转子角速度(rad/s)');
      |     case '2'
      |         disp('获取关节2电机\n外转子角速度(rad/s)');
      |     case '3'
      |         disp('获取关节3电机\n外转子角速度(rad/s)');
      |     case '4'
      |         disp('获取关节4电机\n外转子角速度(rad/s)');
      |     case '5'
      |         disp('获取关节5电机\n外转子角速度(rad/s)');
      |     case '6'
      |         disp('获取关节6电机\n外转子角速度(rad/s)');
      | end
      | color('black');
      | port_label('output', 1, 'Velocity');
      | clear choice1;
  上位机监控窗口1——参数1 : DataStoreWrite  DataStoreName=Send_GUIdata  DataStoreElements=Send_GUIdata(1)
  上位机监控窗口1——参数2 : DataStoreWrite  DataStoreName=Send_GUIdata  DataStoreElements=Send_GUIdata(7)
  上位机监控窗口1——参数3 : DataStoreWrite  DataStoreName=Send_GUIdata  DataStoreElements=Send_GUIdata(13)
  上位机监控窗口2——参数1 : DataStoreWrite  DataStoreName=Send_GUIdata  DataStoreElements=Send_GUIdata(2)
  上位机监控窗口2——参数2 : DataStoreWrite  DataStoreName=Send_GUIdata  DataStoreElements=Send_GUIdata(8)
  上位机监控窗口2——参数3 : DataStoreWrite  DataStoreName=Send_GUIdata  DataStoreElements=Send_GUIdata(14)
  上位机监控窗口3——参数1 : DataStoreWrite  DataStoreName=Send_GUIdata  DataStoreElements=Send_GUIdata(3)
  上位机监控窗口3——参数2 : DataStoreWrite  DataStoreName=Send_GUIdata  DataStoreElements=Send_GUIdata(9)
  上位机监控窗口3——参数3 : DataStoreWrite  DataStoreName=Send_GUIdata  DataStoreElements=Send_GUIdata(15)
  上位机监控窗口4——参数1 : DataStoreWrite  DataStoreName=Send_GUIdata  DataStoreElements=Send_GUIdata(4)
  上位机监控窗口4——参数2 : DataStoreWrite  DataStoreName=Send_GUIdata  DataStoreElements=Send_GUIdata(10)
  上位机监控窗口4——参数3 : DataStoreWrite  DataStoreName=Send_GUIdata  DataStoreElements=Send_GUIdata(16)
  上位机监控窗口5——参数1 : DataStoreWrite  DataStoreName=Send_GUIdata  DataStoreElements=Send_GUIdata(5)
  上位机监控窗口5——参数2 : DataStoreWrite  DataStoreName=Send_GUIdata  DataStoreElements=Send_GUIdata(11)
  上位机监控窗口5——参数3 : DataStoreWrite  DataStoreName=Send_GUIdata  DataStoreElements=Send_GUIdata(17)
  上位机监控窗口6——参数1 : DataStoreWrite  DataStoreName=Send_GUIdata  DataStoreElements=Send_GUIdata(6)
  上位机监控窗口6——参数2 : DataStoreWrite  DataStoreName=Send_GUIdata  DataStoreElements=Send_GUIdata(12)
  上位机监控窗口6——参数3 : DataStoreWrite  DataStoreName=Send_GUIdata  DataStoreElements=Send_GUIdata(18)
  从电机获取到的 各关节的电流 : DataStoreRead  DataStoreName=Motor_Current
  组号1——数据1 : DataStoreRead  DataStoreName=J1  DataStoreElements=J1(1)
  组号1——数据2 : DataStoreRead  DataStoreName=J1  DataStoreElements=J1(2)
  组号1——数据3 : DataStoreRead  DataStoreName=J1  DataStoreElements=J1(3)
  组号1——数据4 : DataStoreRead  DataStoreName=J1  DataStoreElements=J1(4)
  组号1——数据5 : DataStoreRead  DataStoreName=J1  DataStoreElements=J1(5)
  组号1——数据6 : DataStoreRead  DataStoreName=J1  DataStoreElements=J1(6)
  组号2——数据1 : DataStoreRead  DataStoreName=J2  DataStoreElements=J2(1)
  组号2——数据2 : DataStoreRead  DataStoreName=J2  DataStoreElements=J2(2)
  组号2——数据3 : DataStoreRead  DataStoreName=J2  DataStoreElements=J2(3)
  组号2——数据4 : DataStoreRead  DataStoreName=J2  DataStoreElements=J2(4)
  组号2——数据5 : DataStoreRead  DataStoreName=J2  DataStoreElements=J2(5)
  组号2——数据6 : DataStoreRead  DataStoreName=J2  DataStoreElements=J2(6)
  组号3——数据1 : DataStoreRead  DataStoreName=J3  DataStoreElements=J3(1)
  组号3——数据2 : DataStoreRead  DataStoreName=J3  DataStoreElements=J3(2)
  组号3——数据3 : DataStoreRead  DataStoreName=J3  DataStoreElements=J3(3)
  组号3——数据4 : DataStoreRead  DataStoreName=J3  DataStoreElements=J3(4)
  组号3——数据5 : DataStoreRead  DataStoreName=J3  DataStoreElements=J3(5)
  组号3——数据6 : DataStoreRead  DataStoreName=J3  DataStoreElements=J3(6)
  组号4——数据1 : DataStoreRead  DataStoreName=J4  DataStoreElements=J4(1)
  组号4——数据2 : DataStoreRead  DataStoreName=J4  DataStoreElements=J4(2)
  组号4——数据3 : DataStoreRead  DataStoreName=J4  DataStoreElements=J4(3)
  组号4——数据4 : DataStoreRead  DataStoreName=J4  DataStoreElements=J4(4)
  组号4——数据5 : DataStoreRead  DataStoreName=J4  DataStoreElements=J4(5)
  组号4——数据6 : DataStoreRead  DataStoreName=J4  DataStoreElements=J4(6)
  组号5——数据1 : DataStoreRead  DataStoreName=J5  DataStoreElements=J5(1)
  组号5——数据2 : DataStoreRead  DataStoreName=J5  DataStoreElements=J5(2)
  组号5——数据3 : DataStoreRead  DataStoreName=J5  DataStoreElements=J5(3)
  组号5——数据4 : DataStoreRead  DataStoreName=J5  DataStoreElements=J5(4)
  组号5——数据5 : DataStoreRead  DataStoreName=J5  DataStoreElements=J5(5)
  组号5——数据6 : DataStoreRead  DataStoreName=J5  DataStoreElements=J5(6)
  组号6——数据1 : DataStoreRead  DataStoreName=J6  DataStoreElements=J6(1)
  组号6——数据2 : DataStoreRead  DataStoreName=J6  DataStoreElements=J6(2)
  组号6——数据3 : DataStoreRead  DataStoreName=J6  DataStoreElements=J6(3)
  组号6——数据4 : DataStoreRead  DataStoreName=J6  DataStoreElements=J6(4)
  组号6——数据5 : DataStoreRead  DataStoreName=J6  DataStoreElements=J6(4)
  组号6——数据6 : DataStoreRead  DataStoreName=J6  DataStoreElements=J6(6)
  组号7——数据1 : DataStoreRead  DataStoreName=J7  DataStoreElements=J7(1)
  组号7——数据2 : DataStoreRead  DataStoreName=J7  DataStoreElements=J7(2)
  组号7——数据3 : DataStoreRead  DataStoreName=J7  DataStoreElements=J7(3)
  组号7——数据4 : DataStoreRead  DataStoreName=J7  DataStoreElements=J7(4)
  组号7——数据5 : DataStoreRead  DataStoreName=J7  DataStoreElements=J7(5)
  组号7——数据6 : DataStoreRead  DataStoreName=J7  DataStoreElements=J7(6)
  wires:
  从电机获取到的 各关节的电流/1 -> Demux/1

== system DynamicTemplate/GetMotorData ==
  note: 获取关节电流、 角速度、 角度信息
  CANA_284_24 : Subsystem  Priority=4  TreatAsAtomicUnit=on
      settings: RTWSystemCode=Nonreusable function
      mask Display:
      | color('WHITE')
      | disp('JOINT4\n数据读取')
  CANA_285_25 : Subsystem  Priority=5  TreatAsAtomicUnit=on
      settings: RTWSystemCode=Nonreusable function
      mask Display:
      | color('WHITE')
      | disp('JOINT5\n数据读取')
  CANA_286_26 : Subsystem  Priority=6  TreatAsAtomicUnit=on
      settings: RTWSystemCode=Nonreusable function
      mask Display:
      | color('WHITE')
      | disp('JOINT6\n数据读取')
  CANB_281_21 : Subsystem  Priority=1  TreatAsAtomicUnit=on
      settings: RTWSystemCode=Nonreusable function
      mask Display:
      | color('WHITE')
      | disp('JOINT1\n数据读取')
  CANB_282_22 : Subsystem  Priority=2  TreatAsAtomicUnit=on
      settings: RTWSystemCode=Nonreusable function
      mask Display:
      | color('white')
      | disp('JOINT2\n数据读取')
  CANB_283_23 : Subsystem  Priority=3  TreatAsAtomicUnit=on
      settings: RTWSystemCode=Nonreusable function
      mask Display:
      | color('white')
      | disp('JOINT3\n数据读取')

== system DynamicTemplate/SendDataToGUI ==
  note: Upper limit=9
  note: 发送数据给上位机
  note: 定时器步长Fixe-step size=0.001s,
      | 每10ms发送一次数据给上位机
  " " : Subsystem
  Constant : Constant  Value=true  OutDataTypeStr=boolean
  Constant1 : Constant  Value=false  OutDataTypeStr=boolean
  Switch : Switch  Criteria=u2 > Threshold
  广播周期 : simulink/Sources/Counter Limited  uplimit=9  tsamp=-1
  wires:
  Switch/1 -> " "/Enable
  广播周期/1 -> Switch/2
  Constant1/1 -> Switch/1
  Constant/1 -> Switch/3

== system DynamicTemplate/Subsystem ==
  Model Header : Subsystem  mask(Model Header){ShowInLibBrowser=0}
      mask prompts: ShowInLibBrowser "Simulink:masks:CustCodeMaskParam1_MP"
      settings: CopyFcn=cccopyfcn(gcb)  OpenFcn=ccopenfcn('Model Header')
      mask Help: eval('feval(''rtwprivate'',''rtwhelpview'',''rtw_model_header_block'')');
      mask Display: disp('Model\nHeader');
  Model Source : Subsystem  mask(Model Source){ShowInLibBrowser=0}
      mask prompts: ShowInLibBrowser "Simulink:masks:CustCodeMaskParam1_MP"
      settings: CopyFcn=cccopyfcn(gcb)  OpenFcn=ccopenfcn('Model Source')
      mask Help: eval('feval(''rtwprivate'',''rtwhelpview'',''rtw_model_source_block'')');
      mask Display: disp('Model\nSource');
  System Initialize : Subsystem  mask(System Initialize){ShowInLibBrowser=0}
      mask prompts: ShowInLibBrowser "Simulink:masks:CustCodeMaskParam1_MP"
      settings: CopyFcn=cccopyfcn(gcb)  OpenFcn=ccopenfcn('System Initialize Function')
      mask Help: eval('feval(''rtwprivate'',''rtwhelpview'',''rtw_sys_initialize_block'')');
      mask Display: disp('System\nInitialize');

== system DynamicTemplate/接收上位机的数据 ==
  note: 接收上位机数据
  function : TriggerPort  TriggerType=function-call  VariantControl=Variant
  0x0080 : simulink/Logic and Bit Operations/Compare To Constant  relop===  const=hex2dec('0080')  OutDataTypeStr=boolean
  0x88 : simulink/Logic and Bit Operations/Compare To Constant  relop===  const=hex2dec('0088')  OutDataTypeStr=boolean
  Compare To Constant1 : simulink/Logic and Bit Operations/Compare To Constant  relop===  const=hex2dec('0001')  OutDataTypeStr=boolean
  Compare To Constant2 : simulink/Logic and Bit Operations/Compare To Constant  relop===  const=hex2dec('0001')  OutDataTypeStr=boolean
  Data Store Read : DataStoreRead  DataStoreName=PTX
  Data Store Write2 : DataStoreWrite  DataStoreName=StartRobot
  Data Type Conversion : DataTypeConversion  OutDataTypeStr=int16
  Data Type Conversion3 : DataTypeConversion  OutDataTypeStr=double
  Data Type Conversion4 : DataTypeConversion  OutDataTypeStr=uint16
  Demux1 : Demux  Outputs=9
  Logical Operator : Logic  Inputs=4  AllPortsSameDT=off  OutDataTypeStr=boolean
  Mux1 : Mux  Inputs=6
  Subsystem : Subsystem
  Terminator3 : Terminator
  消息使能 : DataStoreMemory  DataStoreName=PTX  ReadBeforeWriteMsg=warning  WriteAfterWriteMsg=warning  WriteAfterReadMsg=warning  InitialValue=true  ShowAdditionalParam=off  OutDataTypeStr=boolean
  获取用户命令 : Subsystem  Priority=1  TreatAsAtomicUnit=on
      settings: RTWSystemCode=Nonreusable function
  wires:
  Compare To Constant2/1 -> Logical Operator/4
  Compare To Constant1/1 -> Logical Operator/3
  Data Store Read/1 -> Logical Operator/2
  Logical Operator/1 -> Data Type Conversion4/1
  0x0080/1 -> Logical Operator/1
  Demux1/4 -> Mux1/2, Compare To Constant2/1
  Demux1/3 -> Mux1/1, Compare To Constant1/1
  Demux1/1 -> 0x0080/1, 0x88/1
  获取用户命令/1(消息) -> Demux1/1
  Demux1/5 -> Mux1/3
  Demux1/6 -> Mux1/4
  Demux1/9 -> Terminator3/1
  Demux1/7 -> Mux1/5
  Demux1/8 -> Mux1/6
  Mux1/1 -> Data Type Conversion/1
  Data Type Conversion/1 -> Data Type Conversion3/1
  Data Type Conversion4/1 -> Data Store Write2/1
  Demux1/2 -> Subsystem/1(组号)
  Data Type Conversion3/1 -> Subsystem/2(数据)
  0x88/1 -> Subsystem/Enable

== system DynamicTemplate/DynamicsController/DriveMotor ==
  Tau1 : Inport
  Tau2 : Inport  Port=2
  Tau3 : Inport  Port=3
  Tau4 : Inport  Port=4
  Tau5 : Inport  Port=5
  Tau6 : Inport  Port=6
  Enable : Inport  Port=7
  BottomDriver : Subsystem
  Data Store Memory1 : DataStoreMemory  DataStoreName=TXD  ReadBeforeWriteMsg=warning  WriteAfterWriteMsg=warning  WriteAfterReadMsg=warning  InitialValue=[0]  ShowAdditionalParam=off  OutDataTypeStr=uint8
      settings: RTWStateStorageClass=ExportedGlobal
  Data Store Read4 : DataStoreRead  DataStoreName=TXD
  Saturation{1..6} (6 alike) : Saturate  UpperLimit=900  LowerLimit=-900
  驱动器指令 : Subsystem  TreatAsAtomicUnit=on
      settings: RTWSystemCode=Nonreusable function
  wires:
  Data Store Read4/1 -> BottomDriver/Enable
  驱动器指令/4(MSG4) -> BottomDriver/4(JOINT4)
  驱动器指令/3(MSG3) -> BottomDriver/3(JOINT3)
  驱动器指令/1(MSG1) -> BottomDriver/1(JOINT1)
  驱动器指令/2(MSG2) -> BottomDriver/2(JOINT2)
  Enable/1 -> 驱动器指令/7(Enable)
  驱动器指令/5(MSG5) -> BottomDriver/5(JOINT5)
  Saturation2/1 -> 驱动器指令/1(Current1)
  Saturation1/1 -> 驱动器指令/2(Current2)
  Saturation3/1 -> 驱动器指令/3(Current3)
  Saturation4/1 -> 驱动器指令/4(Current4)
  Saturation5/1 -> 驱动器指令/5(Current5)
  Tau1/1 -> Saturation2/1
  Tau2/1 -> Saturation1/1
  Tau3/1 -> Saturation3/1
  Tau4/1 -> Saturation4/1
  Tau5/1 -> Saturation5/1
  驱动器指令/6(MSG6) -> BottomDriver/6(JOINT6)
  Tau6/1 -> Saturation6/1
  Saturation6/1 -> 驱动器指令/6(Current6)
